simulink model "openLoopModel"  (R2018a)
settings: Solver=VariableStepAuto  StartTime=0.0  StopTime=15  RelTol=1e-3
settings Model: Creator=diogo  LastModifiedBy=diogo

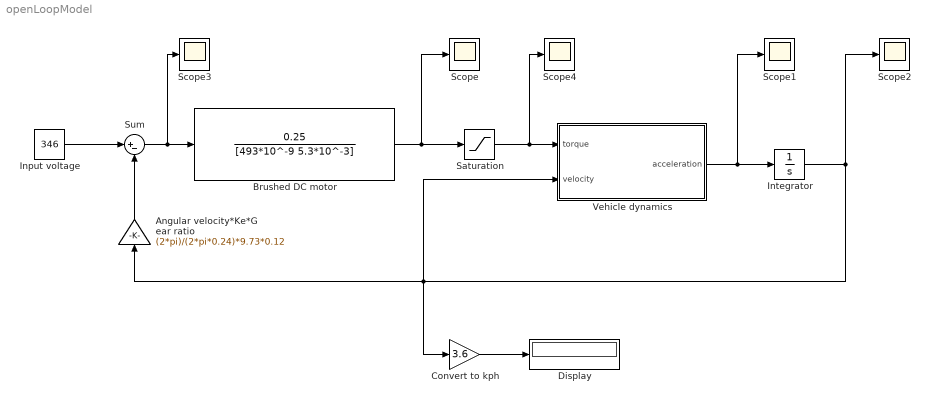
== system openLoopModel ==
  Angular velocity*Ke*Gear ratio : Gain  Gain=(2*pi)/(2*pi*0.24)*9.73*0.12
  Brushed DC motor : TransferFcn  Numerator=[0.25]  Denominator=[493*10^-9 5.3*10^-3]
  Convert to kph : Gain  Gain=3.6
  Display : Display
  Input voltage : Constant  Value=346
  Integrator : Integrator
  Saturation : Saturate  UpperLimit=601  LowerLimit=0
  Scope{,1..4} (5 alike) : Scope
  Sum : Sum  Inputs=|+-
  Vehicle dynamics : MATLAB Function  TreatAsAtomicUnit=on
  wires:
  Input voltage/1 -> Sum/1
  Angular velocity*Ke*Gear ratio/1 -> Sum/2
  Sum/1 -> Brushed DC motor/1, Scope3/1
  Brushed DC motor/1 -> Scope/1, Saturation/1
  Vehicle dynamics/1(acceleration) -> Scope1/1, Integrator/1
  Integrator/1 -> Angular velocity*Ke*Gear ratio/1, Vehicle dynamics/2(velocity), Convert to kph/1, Scope2/1
  Convert to kph/1 -> Display/1
  Saturation/1 -> Scope4/1, Vehicle dynamics/1(torque)

== matlab function openLoopModel/Vehicle dynamics ==
  data: torque input; acceleration output; velocity input
function acceleration = fcn(torque, velocity)
acceleration = (40.5*torque*0.6 - 413 - 0.3381*velocity^2)/2108;
